simulink model "ELEC367SIMULINKPROJECT"  (R2024b)
settings: Solver=VariableStepAuto  StartTime=0.0  StopTime=60  RelTol=1e-3
settings Model: Creator=mohdm  LastModifiedBy=mohdm

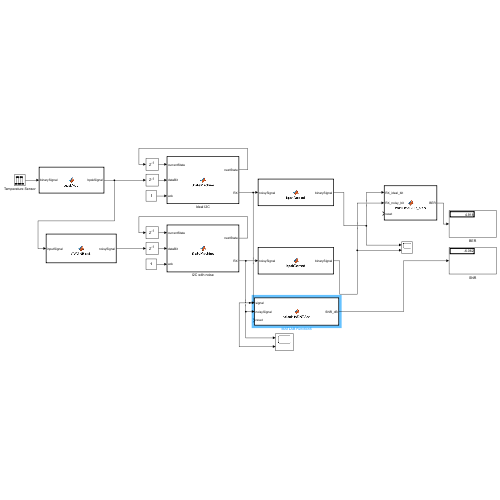
[thumbnail: Simulink's stored preview of the top-level diagram]
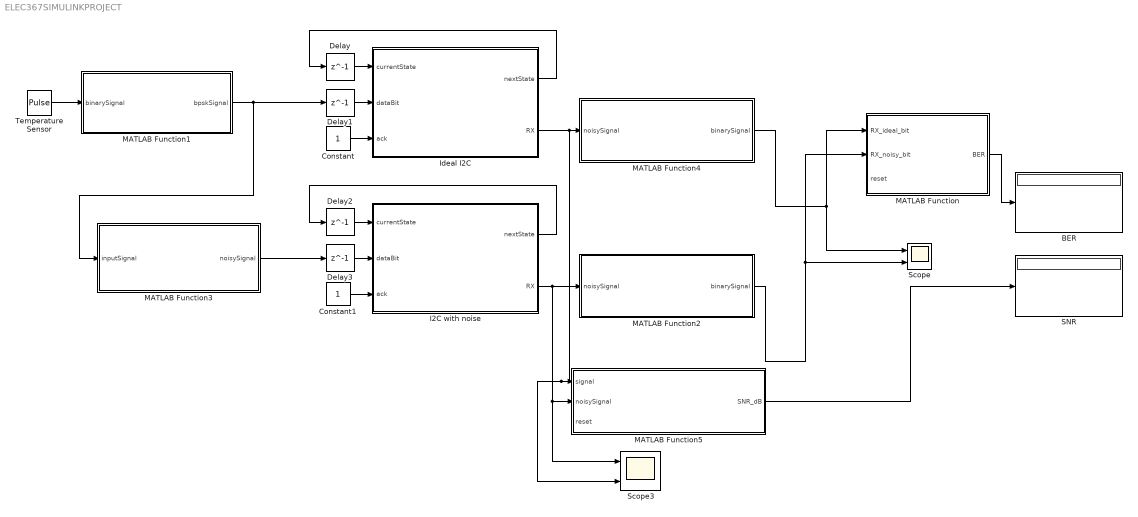
== system ELEC367SIMULINKPROJECT ==
  BER : Display
  Constant : Constant
  Constant1 : Constant
  Delay{,1..3} (4 alike) : Delay  DelayLength=1  InitialCondition=0
  I2C with noise : MATLAB Function  TreatAsAtomicUnit=on
  Ideal I2C : MATLAB Function  TreatAsAtomicUnit=on
  MATLAB Function : MATLAB Function  TreatAsAtomicUnit=on
  MATLAB Function1 : MATLAB Function  TreatAsAtomicUnit=on
  MATLAB Function2 : MATLAB Function  TreatAsAtomicUnit=on
  MATLAB Function3 : MATLAB Function  TreatAsAtomicUnit=on
  MATLAB Function4 : MATLAB Function  TreatAsAtomicUnit=on
  MATLAB Function5 : MATLAB Function  TreatAsAtomicUnit=on
  SNR : Display
  Scope : Scope  NumInputPorts=2
  Scope3 : Scope  NumInputPorts=2
  Temperature Sensor : DiscretePulseGenerator  Period=10  PulseWidth=5
  wires:
  Delay/1 -> Ideal I2C/1(currentState)
  Ideal I2C/1(nextState) -> Delay/1
  Delay1/1 -> Ideal I2C/2(dataBit)
  Delay3/1 -> I2C with noise/2(dataBit)
  Delay2/1 -> I2C with noise/1(currentState)
  I2C with noise/1(nextState) -> Delay2/1
  Ideal I2C/2(RX) -> Scope3/2, MATLAB Function5/1(signal), MATLAB Function4/1(noisySignal)
  I2C with noise/2(RX) -> Scope3/1, MATLAB Function5/2(noisySignal), MATLAB Function2/1(noisySignal)
  Temperature Sensor/1 -> MATLAB Function1/1(binarySignal)
  MATLAB Function/1(BER) -> BER/1
  Constant/1 -> Ideal I2C/3(ack)
  Constant1/1 -> I2C with noise/3(ack)
  MATLAB Function1/1(bpskSignal) -> MATLAB Function3/1(inputSignal), Delay1/1
  MATLAB Function2/1(binarySignal) -> MATLAB Function/2(RX_noisy_bit), Scope/2
  MATLAB Function4/1(binarySignal) -> MATLAB Function/1(RX_ideal_bit), Scope/1
  MATLAB Function3/1(noisySignal) -> Delay3/1
  MATLAB Function5/1(SNR_dB) -> SNR/1

== matlab function ELEC367SIMULINKPROJECT/I2C with noise ==
  data: currentState input; nextState output; dataBit input; RX output; ack input
function [nextState, RX] = StateMachine(currentState, dataBit,ack)
RX = 0;
switch currentState
    case 1 %Idle 
            nextState = 2; %Start

    case 2 % Start
            nextState = 3; %Address

    case 3 %Address 
            slaveAddress = 80;
            nextState = 4;
    case 4 %%ACK
        if ack == true
            nextState = 5;
        else 
            nextState = 2;
        end
    case 5 %TX
        RX = dataBit;
        nextState = 6;
    case 6 % STOP
        nextState = 1;
    otherwise 
        nextState = 1;
end

== matlab function ELEC367SIMULINKPROJECT/Ideal I2C ==
  data: currentState input; nextState output; dataBit input; RX output; ack input
function [nextState, RX] = StateMachine(currentState, dataBit,ack)
RX = 0;
switch currentState
    case 1 %Idle 
            nextState = 2; %Start

    case 2 % Start
            nextState = 3; %Address

    case 3 %Address 
            slaveAddress = 80;
            nextState = 4;
    case 4 %%ACK
        if ack== true
            nextState = 5;
        else 
            nextState = 2;
        end
    case 5 %TX
        RX = dataBit;
        nextState = 6;
    case 6 % STOP
        nextState = 1;
    otherwise 
        nextState = 1;
end

== matlab function ELEC367SIMULINKPROJECT/MATLAB Function ==
  data: RX_ideal_bit input; BER output; RX_noisy_bit input; reset input
function BER = calculateBER_step(RX_ideal_bit, RX_noisy_bit, reset)
    % Function to calculate BER with optional reset
    persistent totalBits numErrors

    % Initialize or reset persistent variables
    if isempty(totalBits) || reset
        totalBits = 0; % Initialize or reset total bits
        numErrors = 0; % Initialize or reset error count
    end

    % Ensure inputs are logical
    RX_ideal_bit = logical(RX_ideal_bit);
    RX_noisy_bit = logical(RX_noisy_bit);

    % Update counters
    if isscalar(RX_ideal_bit) && isscalar(RX_noisy_bit)
        % Single-bit case
        totalBits = totalBits + 1;
        numErrors = numErrors + (RX_ideal_bit ~= RX_noisy_bit);
    else
        % Multi-bit case (if signals are vectors)
        totalBits = totalBits + length(RX_ideal_bit);
        numErrors = numErrors + sum(RX_ideal_bit ~= RX_noisy_bit);
    end

    % Calculate BER
    if totalBits > 0
        BER = (numErrors / totalBits) * 100; % BER as a percentage
    else
        BER = 0;
    end

   % Debugging Outputs
coder.extrinsic('sprintf', 'disp'); % Declare sprintf and disp as extrinsic

% Convert logical RX bits to numeric for printing
RX_ideal_numeric = double(RX_ideal_bit); % Convert to 0 or 1
RX_noisy_numeric = double(RX_noisy_bit); % Convert to 0 or 1

% Create a debug string with RX bits included
debugStr = sprintf('Total Bits: %d, Errors: %d, BER: %.5f%%, RX Ideal: %d, RX Noisy: %d', ...
                   totalBits, numErrors, BER, RX_ideal_numeric, RX_noisy_numeric);

% Display debugging information
disp(debugStr); % Print to Command Window

end

== matlab function ELEC367SIMULINKPROJECT/MATLAB Function1 ==
  data: binarySignal input; bpskSignal output
function bpskSignal = bpskMod(binarySignal)
    % BPSK Modulation
    % binarySignal: Input binary signal (0s and 1s)
    % bpskSignal: Output BPSK modulated signal (-1s and 1s)
    
    bpskSignal = 2 * binarySignal - 1; % Map 0 -> -1 and 1 -> 1
end

== matlab function ELEC367SIMULINKPROJECT/MATLAB Function2 ==
  data: noisySignal input; binarySignal output
function binarySignal = bpskDemod(noisySignal)
    % BPSK Demodulation
    % noisySignal: Noisy BPSK signal
    % binarySignal: Recovered binary signal (0s and 1s)
    
    binarySignal = noisySignal > 0; % Compare to 0, map >0 -> 1, <=0 -> 0
end

== matlab function ELEC367SIMULINKPROJECT/MATLAB Function3 ==
  data: inputSignal input; noisySignal output
function noisySignal = AWGNBlock(inputSignal)
    % AWGNBlock - Adds Additive White Gaussian Noise to a signal
    %
    % Inputs:
    %   inputSignal - Input signal (vector or scalar)
    %
    % Output:
    %   noisySignal - Signal with AWGN applied

    % Set the SNR (Signal-to-Noise Ratio in dB)
    snr = -5; % Adjust this value as needed

    % Ensure input is a double
    inputSignal = double(inputSignal);

    % Calculate signal power
    signalPower = mean(inputSignal.^2);

    % Calculate noise power based on the SNR
    noisePower = signalPower / (10^(snr / 10));

    % Generate Gaussian noise with zero mean and the calculated variance
    noise = sqrt(noisePower) * randn(size(inputSignal));

    % Add noise to the input signal
    noisySignal = inputSignal + noise;
end

== matlab function ELEC367SIMULINKPROJECT/MATLAB Function4 ==
  data: noisySignal input; binarySignal output
function binarySignal = bpskDemod(noisySignal)
    % BPSK Demodulation
    % noisySignal: Noisy BPSK signal
    % binarySignal: Recovered binary signal (0s and 1s)
    
    binarySignal = noisySignal > 0; % Compare to 0, map >0 -> 1, <=0 -> 0
end

== matlab function ELEC367SIMULINKPROJECT/MATLAB Function5 ==
  data: signal input; SNR_dB output; noisySignal input; reset input
function SNR_dB = calculateSNRAcc(signal, noisySignal, reset)
    % Function to calculate SNR over time by accumulating values
    % Inputs:
    % - signal: Ideal signal (reference signal)
    % - noisySignal: Received signal with noise
    % - reset: Boolean to reset accumulated values
    % Output:
    % - SNR_dB: Signal-to-Noise Ratio in dB

    % Persistent arrays for signal power and noise power
    persistent signalPowerArray noisePowerArray

    % Reset or initialize persistent variables
    if isempty(signalPowerArray) || reset
        signalPowerArray = [];
        noisePowerArray = [];
    end

    % Calculate current signal and noise powers
    currentSignalPower = mean(abs(signal).^2); % Instantaneous signal power
    noise = noisySignal - signal;
    currentNoisePower = mean(abs(noise).^2); % Instantaneous noise power

    % Append to persistent arrays
    signalPowerArray = [signalPowerArray; currentSignalPower];
    noisePowerArray = [noisePowerArray; currentNoisePower];

    % Calculate accumulated signal and noise powers
    totalSignalPower = mean(signalPowerArray); % Average signal power
    totalNoisePower = mean(noisePowerArray);   % Average noise power

    % Calculate SNR in dB
    if totalNoisePower > 0
        SNR_dB = 10 * log10(totalSignalPower / totalNoisePower);
    else
        SNR_dB = Inf; % Infinite SNR if noise power is zero
    end

    % Debugging Outputs
    coder.extrinsic('sprintf', 'disp'); % Allow sprintf and disp in Simulink
    debugStr = sprintf('Signal Power: %.5f, Noise Power: %.5f, SNR (dB): %.5f', ...
                        totalSignalPower, totalNoisePower, SNR_dB);
    disp(debugStr); % Print debugging information
end
